simulink model "re_written_control_system"  (R2024b)
settings: Solver=VariableStepAuto  StartTime=0.0  StopTime=5000  RelTol=1e-3
InitFcn:
  | [moter_left, moter_right, moter_bow, A ,mass, boat_dimensions, friction, inertia, wind_gain] = get_parameters()
  | [K, B, thuster_angle] = re_LQR()
values from neighbouring files (symbols this model uses):
  A = [bx/m 0 0 ... (first row only)    [calculateLQR.m]    (also in extended_kalman_filter_sim_2.m = [0 0 0 1 0 0 0 0 0; 0 0 0 0 1 0 0 0 0; 0 0 0 0 0 1 0 0 0; 0 ; get_parameters.m = [b_x/mass 0        0; h_inf.m = [0, 1, 0; kalman_filter_sim.m = [0, 1, 0 ; 0, (b+bc)/m, 0 ;0, 0,    0])
  B = B_fuc(thuster_angle)    [LQR.m]    (also in calculateLQR.m = [cos(theta_right+vector_angel_1), cos(theta_left+vector_ange; h_inf.m = [0, 0, 0; kalman_filter_sim.m = [0, 0, 0; 0, 1/m, 0; 0, 0, 0]; kalman_filter_sim_2.m = [0; 1/m; 0])
  boat_dimensions = [length_x, length_y ,length_z]    [get_parameters.m]
  friction = [b_x, b_y, b_t]    [get_parameters.m]
  inertia = (length_y^2+length_x^2)*mass*1/12    (= 8952.5)    [get_parameters.m]
  K = Pm*H'*inv(H*Pm*H'+R)    [extended_kalman_filter_sim.m]    (also in extended_kalman_filter_sim_2.m = Pm * H' / (H * Pm * H' + M * R * M'); h_inf.m = Pm * L / (I + H * Pm * L); kalman_filter_sim.m; ll.m = P*H'/S)
  mass = 3000+r    (= 3000)    [get_parameters.m]
  moter_bow = [ 0,           length_y+c  , 0, 0]    [extended_kalman_filter_sim_2.m]    (also in get_parameters.m = [ 0,             length_y-r, 0, 0])
  moter_left = [-length_x/2, -length_y/2+c, 0, 0]    [extended_kalman_filter_sim_2.m]    (also in get_parameters.m = [-length_x/2, -length_y/2+r, 0, 0])
  moter_right = [ length_x/2, -length_y/2+c, 0, 0]    [extended_kalman_filter_sim_2.m]    (also in get_parameters.m = [ length_x/2, -length_y/2+r, 0, 0])
  thuster_angle = [thuster_angle, 0]    [LQR.m]    (also in re_LQR.m)
  wind_gain = 0    [get_parameters.m]
settings Model: Creator=klyx  LastModifiedBy=klyx

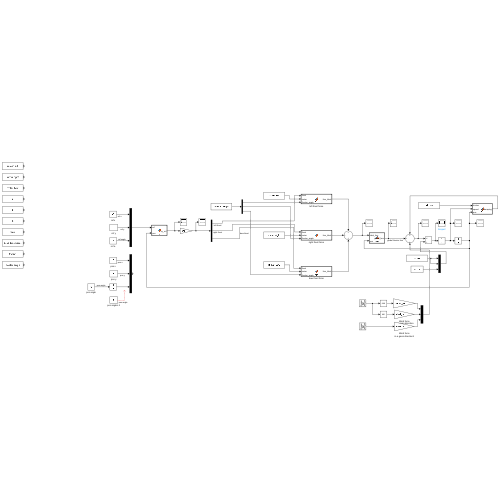
[thumbnail: Simulink's stored preview of the top-level diagram]
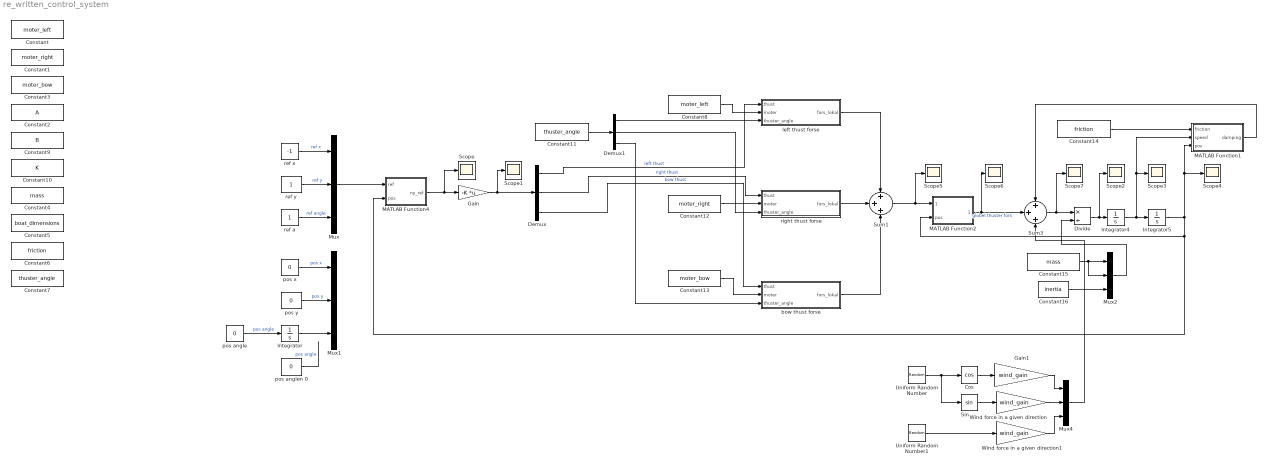
== system re_written_control_system ==
  Constant : Constant  Value=moter_left
  Constant1 : Constant  Value=moter_right
  Constant10 : Constant  Value=K
  Constant11 : Constant  Value=thuster_angle
  Constant12 : Constant  Value=moter_right
  Constant13 : Constant  Value=moter_bow
  Constant14 : Constant  Value=friction
  Constant15 : Constant  Value=mass
  Constant16 : Constant  Value=inertia
  Constant2 : Constant  Value=A
  Constant3 : Constant  Value=moter_bow
  Constant4 : Constant  Value=mass
  Constant5 : Constant  Value=boat_dimensions
  Constant6 : Constant  Value=friction
  Constant7 : Constant  Value=thuster_angle
  Constant8 : Constant  Value=moter_left
  Constant9 : Constant  Value=B
  Cos : Trigonometry  Operator=cos
  Demux : Demux  Outputs=3
  Demux1 : Demux  Outputs=3
  Divide : Product  Inputs=*/
  Gain : Gain  Gain=-K  Multiplication=Matrix(K*u)
  Gain1 : Gain  Gain=wind_gain
  Integrator : Integrator
  Integrator4 : Integrator  InitialCondition=[0; 0; 0]
  Integrator5 : Integrator  InitialCondition=[0; 0; 0]
  MATLAB Function1 : MATLAB Function  TreatAsAtomicUnit=on
  MATLAB Function2 : MATLAB Function  TreatAsAtomicUnit=on
  MATLAB Function4 : MATLAB Function  TreatAsAtomicUnit=on
  Mux{,1..2,4} (4 alike) : Mux  Inputs=3
  Scope{,1..7} (8 alike) : Scope
  Sin : Trigonometry
  Sum1 : Sum  Inputs=+++
  Sum3 : Sum  Inputs=+++
  Uniform Random Number : UniformRandomNumber  Minimum=0  Maximum=6.28  Seed=55  SampleTime=1
  Uniform Random Number1 : UniformRandomNumber  Minimum=-6.28  Maximum=6.28  Seed=8965  SampleTime=1
  Wind force in a given direction : Gain  Gain=wind_gain
  Wind force in a given direction1 : Gain  Gain=wind_gain
  bow thust forse : MATLAB Function  TreatAsAtomicUnit=on
  left thust forse : MATLAB Function  TreatAsAtomicUnit=on
  pos angle : Constant  Value=0
  pos anglen 0 : Constant  Value=0
  pos x : Constant  Value=0
  pos y : Constant  Value=0
  ref a : Constant
  ref x : Constant  Value=-1
  ref y : Constant
  right thust forse : MATLAB Function  TreatAsAtomicUnit=on
  wires:
  ref x/1 -> Mux/1  "ref x"
  ref y/1 -> Mux/2  "ref y"
  ref a/1 -> Mux/3  "ref angle"
  pos y/1 -> Mux1/2  "pos y"
  pos x/1 -> Mux1/1  "pos x"
  pos angle/1 -> Integrator/1  "pos angle"
  MATLAB Function4/1(ny_ref) -> Scope/1, Gain/1
  pos anglen 0/1 -> ?  "pos angle"
  Integrator/1 -> Mux1/3
  Gain/1 -> Scope1/1, Demux/1
  Demux/1 -> left thust forse/1(thust)  "left thust"
  Demux/3 -> bow thust forse/1(thust)  "bow thust"
  Constant8/1 -> left thust forse/2(moter)
  Constant11/1 -> Demux1/1
  Demux1/1 -> left thust forse/3(thuster_angle)
  Constant13/1 -> bow thust forse/2(moter)
  Demux/2 -> right thust forse/1(thust)  "right thust"
  Demux1/3 -> bow thust forse/3(thuster_angle)
  Constant12/1 -> right thust forse/2(moter)
  Demux1/2 -> right thust forse/3(thuster_angle)
  Integrator5/1 -> Scope4/1, MATLAB Function1/3(pos), MATLAB Function2/2(pos), MATLAB Function4/2(pos)
  Constant15/1 -> Mux2/2, Mux2/1
  Sum1/1 -> MATLAB Function2/1(lokal_fors), Scope5/1
  Integrator4/1 -> Integrator5/1, Scope3/1, MATLAB Function1/2(speed)
  Mux2/1 -> Divide/2
  Divide/1 -> Scope2/1, Integrator4/1
  Constant16/1 -> Mux2/3
  MATLAB Function1/1(damping) -> Sum3/1
  Sum3/1 -> Scope7/1, Divide/1
  Constant14/1 -> MATLAB Function1/1(friction)
  MATLAB Function2/1(globel_fors) -> Scope6/1, Sum3/2  "globel thuster fors"
  Mux/1 -> MATLAB Function4/1(ref)
  Uniform Random Number/1 -> Sin/1, Cos/1
  Cos/1 -> Gain1/1
  Sin/1 -> Wind force in a given direction/1
  Uniform Random Number1/1 -> Wind force in a given direction1/1
  Gain1/1 -> Mux4/1
  Wind force in a given direction/1 -> Mux4/2
  Wind force in a given direction1/1 -> Mux4/3
  Mux4/1 -> Sum3/3
  right thust forse/1(fors_lokal) -> Sum1/2
  left thust forse/1(fors_lokal) -> Sum1/1
  bow thust forse/1(fors_lokal) -> Sum1/3

== matlab function re_written_control_system/MATLAB Function1 ==
  data: friction input; damping output; speed input; pos input
function damping = fcn(friction, speed, pos)

firk = [friction(1) 0           0           ;
        0           friction(2) 0           ;
        0           0           friction(3)];

glo_to_lok = [cos(-pos(3)) -sin(-pos(3)) 0 ;
              sin(-pos(3)) cos(-pos(3))  0 ;
              0           0              1]

%s = speed
rotl = inv(glo_to_lok)*firk*glo_to_lok;
damping = inv(glo_to_lok)*firk*glo_to_lok*speed;

== matlab function re_written_control_system/MATLAB Function4 ==
  data: ref input; ny_ref output; pos input
function ny_ref = fcn(ref ,pos)

xy_pos = [0 0 ref(1);
          0 0 ref(2);
          0 0 1];

glo_to_lok = [cos(pos(3)) -sin(pos(3)) pos(1);
              sin(pos(3)) cos(pos(3))  pos(2);
              0           0            1];


lok_ref = inv(glo_to_lok)*xy_pos;

ny_ref  = [pos(1) - lok_ref(1,3); pos(2) - lok_ref(2,3); pos(3) - ref(3)];

== matlab function re_written_control_system/bow thust forse ==
  data: thust input; fors_lokal output; moter input; thuster_angle input
function fors_lokal  = fcn(thust, moter, thuster_angle)
%this is the in the boat local frame
Fx     = cos(thuster_angle)*thust;
Fy     = sin(thuster_angle)*thust;
torque = sin(moter(3)+thuster_angle)*moter(4)*thust;
fors_lokal = [Fx, Fy, torque];

== matlab function re_written_control_system/left thust forse ==
  data: thust input; fors_lokal output; moter input; thuster_angle input
function fors_lokal = fcn(thust, moter, thuster_angle)
%this is the in the boat local frame
Fx     = cos(thuster_angle)*thust;
Fy     = sin(thuster_angle)*thust;
torque = sin(moter(3)+thuster_angle)*moter(4)*thust;
fors_lokal = [Fx, Fy, torque];

== matlab function re_written_control_system/MATLAB Function2 ==
  data: lokal_fors input; globel_fors output; pos input
function globel_fors = fcn(lokal_fors ,pos)

xy_pos = [lokal_fors(1);lokal_fors(2)];

glo_to_lok = [cos(pos(3)) -sin(pos(3));
              sin(pos(3)) cos(pos(3))];

gb_xy_fors = glo_to_lok*xy_pos;

globel_fors  = [gb_xy_fors(1);gb_xy_fors(2); lokal_fors(3)];

== matlab function re_written_control_system/right thust forse ==
  data: thust input; fors_lokal output; moter input; thuster_angle input
function fors_lokal  = fcn(thust, moter, thuster_angle)
%this is the in the boat local frame
Fx     = cos(thuster_angle)*thust;
Fy     = sin(thuster_angle)*thust;
torque = sin(moter(3)+thuster_angle)*moter(4)*thust;
fors_lokal = [Fx, Fy, torque];
